simulink model "N3Z_tonetestprevious"  (R2014b)
settings: Solver=ode3  SolverMode=SingleTasking  StartTime=0.0  StopTime=1e-4  FixedStep=fpgaclk  RelTol=1e-3
PreLoadFcn:
  | %fpgaclk=1/32.768e6
  | fpgaclk=1/49.162e6
  | 
  | SerialData=[1,zeros(1,11),1,0,0,1]
  | load ../N3workingG/window
  | win=win';  %Go back to using flatter and wider windowed sync function
  | %load ../N3workingG/hanning    %use Hahn window
  | 
  | load ../N3workingG/PREemphasis   %For pre-empasis and deemphasis FIRs
  | 
  | %LUT3=xls2LUT2('../IQI_Qdemod.xls'); LUT3
  | load ../N3workingG/LUT3
  | load ../N3workingG/FIRiq2
  | % xls2LUT
  | 
  | GetProgFiles
  | 
  | PinAssignments    %Get Pin references for TE0722
  | 
  | 
  | 
  | 
  | 
  | %LCD
  | LCDdata=[LCD_D7,LCD_D6,LCD_D5,LCD_D4,LCD_D3,LCD_D2,LCD_D1,LCD_D0] %Note MSB...LSB!
  | LCDctrl=[LCD_E,LCD_RW,LCD_RS];
  | 
  | %for RS232 on pins 3 and 5 of USBB
  | 
  | %BT chip connections for WT12
  | 
  | RX_BT=RXD
  | TX_BT=TXD
  | 
  | RST_BB=RES
  | 
  | %PCMC=PCMC
  | %PCMS=PCMS
  | %PCMI=PCMI
  | %PCMO=PCMO
  | 
  | %Aliases:
  | SRDBT=PCMI
  | STDBT=PCMO
  | SCLK_BT=PCMC
  | SFS_BT=PCMS
  | 
  | %ADC control
  | 
  | %SDOA=SDOA
  | %SDOB=SDOB
  | %SCK=SCK
  | CONV=Csbar
  | CAL=Cal
  | 
  | ADC_G=[ADC_G3,ADC_G2,ADC_G1,ADC_G0]
  | %PD settings hard coded now
  | 
  | %%%%%%
  | TX_LOW=TX_Low
  | ... (+11 lines)
StartFcn:
  | SerialData=[1,zeros(1,11),1,0,0,1]
values from neighbouring files (symbols this model uses):
  ADC_G0 = {'P10'}    [PinAssignments.m]
  ADC_G1 = {'P11'}    [PinAssignments.m]
  ADC_G2 = {'N14'}    [PinAssignments.m]
  ADC_G3 = {'M11'}    [PinAssignments.m]
  Cal = {'L12'}    [PinAssignments.m]
  Csbar = {'M12'}    [PinAssignments.m]
  LCD_D0 = {'J13'}    [PinAssignments.m]
  LCD_D1 = {'J14'}    [PinAssignments.m]
  LCD_D2 = {'F15'}    [PinAssignments.m]
  LCD_D3 = {'H14'}    [PinAssignments.m]
  LCD_D4 = {'G12'}    [PinAssignments.m]
  LCD_D5 = {'L15'}    [PinAssignments.m]
  LCD_D6 = {'M14'}    [PinAssignments.m]
  LCD_D7 = {'K15'}    [PinAssignments.m]
  PCMC = {'H11'}    [PinAssignments.m]
  PCMI = {'H12'}    [PinAssignments.m]
  PCMO = {'N13'}    [PinAssignments.m]
  PCMS = {'M10'}    [PinAssignments.m]
  RES = {'G11'}    [PinAssignments.m]
  RXD = {'H13'}    [PinAssignments.m]
  TX_Low = {'P15'}    [PinAssignments.m]
  TXD = {'P13'}    [PinAssignments.m]
undefined symbols (not defined in the file or in its folder): AXI4, FIRRX, FIRTX, Lite
libraries: xbsIndex_r4 x1250, MyFunctions x43
(part 7 of 10)

== system N3Z_tonetestprevious/DSProcessor1/OutputRegister/Subsystem11 ==
  Data : Inport
  PortId : Inport  Port=2
  Write : Inport  Port=3
  Logical : xbsIndex_r4/Logical  logical_function=AND  inputs=2  en=off  latency=0  precision=Full  arith_type=Unsigned  n_bits=8  bin_pt=2  align_bp=on  dbl_ovrd=off  block_type=logical
      settings: xl_area=[1 0 0 1 0 0 0]  block_version=VER_STRING_GOES_HERE
  PortAddress : xbsIndex_r4/Constant  const=11  gui_display_data_type=Fixed-point  arith_type=Unsigned  n_bits=8  bin_pt=0  preci_type=Single  exp_width=8  frac_width=24  explicit_period=on  period=fpgaclk  equ=P=C  opselect=C  inp2=PCIN>>17  opr=+  inp1=P  carry=CIN  dbl_ovrd=off  block_type=constant
      settings: block_version=VER_STRING_GOES_HERE
  Register1 : xbsIndex_r4/Register  init=151  rst=off  en=on  dbl_ovrd=off  block_type=register
      settings: xl_area=[4 8 0 0 0 0 0]  block_version=VER_STRING_GOES_HERE
  Relational1 : xbsIndex_r4/Relational  mode=a=b  op_type=Bool  en=off  latency=0  dbl_ovrd=off  block_type=relational
      settings: xl_area=[2 0 0 4 0 0 0]  block_version=VER_STRING_GOES_HERE
  LatchedData : Outport
  wires:
  Relational1/1 -> Logical/1
  Logical/1 -> Register1/2
  PortAddress/1 -> Relational1/2
  Data/1 -> Register1/1
  PortId/1 -> Relational1/1
  Write/1 -> Logical/2
  Register1/1 -> LatchedData/1

== system N3Z_tonetestprevious/DSProcessor1/OutputRegister/Subsystem12 ==
  Data : Inport
  PortId : Inport  Port=2
  Write : Inport  Port=3
  Logical : xbsIndex_r4/Logical  logical_function=AND  inputs=2  en=off  latency=0  precision=Full  arith_type=Unsigned  n_bits=8  bin_pt=2  align_bp=on  dbl_ovrd=off  block_type=logical
      settings: xl_area=[1 0 0 1 0 0 0]  block_version=VER_STRING_GOES_HERE
  PortAddress : xbsIndex_r4/Constant  const=12  gui_display_data_type=Fixed-point  arith_type=Unsigned  n_bits=8  bin_pt=0  preci_type=Single  exp_width=8  frac_width=24  explicit_period=on  period=fpgaclk  equ=P=C  opselect=C  inp2=PCIN>>17  opr=+  inp1=P  carry=CIN  dbl_ovrd=off  block_type=constant
      settings: block_version=VER_STRING_GOES_HERE
  Register1 : xbsIndex_r4/Register  init=151  rst=off  en=on  dbl_ovrd=off  block_type=register
      settings: xl_area=[4 8 0 0 0 0 0]  block_version=VER_STRING_GOES_HERE
  Relational1 : xbsIndex_r4/Relational  mode=a=b  op_type=Bool  en=off  latency=0  dbl_ovrd=off  block_type=relational
      settings: xl_area=[2 0 0 4 0 0 0]  block_version=VER_STRING_GOES_HERE
  LatchedData : Outport
  Ack_Fifo : Outport  Port=2
  wires:
  Relational1/1 -> Logical/1
  Logical/1 -> Register1/2, Ack_Fifo/1
  PortAddress/1 -> Relational1/2
  Data/1 -> Register1/1
  PortId/1 -> Relational1/1
  Write/1 -> Logical/2
  Register1/1 -> LatchedData/1

== system N3Z_tonetestprevious/DSProcessor1/OutputRegister/Subsystem13 ==
  Data : Inport
  PortId : Inport  Port=2
  Write : Inport  Port=3
  Logical : xbsIndex_r4/Logical  logical_function=AND  inputs=2  en=off  latency=0  precision=Full  arith_type=Unsigned  n_bits=8  bin_pt=2  align_bp=on  dbl_ovrd=off  block_type=logical
      settings: xl_area=[1 0 0 1 0 0 0]  block_version=VER_STRING_GOES_HERE
  PortAddress : xbsIndex_r4/Constant  const=13  gui_display_data_type=Fixed-point  arith_type=Unsigned  n_bits=8  bin_pt=0  preci_type=Single  exp_width=8  frac_width=24  explicit_period=on  period=fpgaclk  equ=P=C  opselect=C  inp2=PCIN>>17  opr=+  inp1=P  carry=CIN  dbl_ovrd=off  block_type=constant
      settings: block_version=VER_STRING_GOES_HERE
  Register1 : xbsIndex_r4/Register  init=0  rst=off  en=on  dbl_ovrd=off  block_type=register
      settings: xl_area=[4 8 0 0 0 0 0]  block_version=VER_STRING_GOES_HERE
  Relational1 : xbsIndex_r4/Relational  mode=a=b  op_type=Bool  en=off  latency=0  dbl_ovrd=off  block_type=relational
      settings: xl_area=[2 0 0 4 0 0 0]  block_version=VER_STRING_GOES_HERE
  LatchedData : Outport
  NewValue : Outport  Port=2
  wires:
  Relational1/1 -> Logical/1
  Logical/1 -> Register1/2, NewValue/1
  PortAddress/1 -> Relational1/2
  Data/1 -> Register1/1
  PortId/1 -> Relational1/1
  Write/1 -> Logical/2
  Register1/1 -> LatchedData/1

== system N3Z_tonetestprevious/DSProcessor1/OutputRegister/Subsystem14 ==
  Data : Inport
  PortId : Inport  Port=2
  Write : Inport  Port=3
  Logical : xbsIndex_r4/Logical  logical_function=AND  inputs=2  en=off  latency=0  precision=Full  arith_type=Unsigned  n_bits=8  bin_pt=2  align_bp=on  dbl_ovrd=off  block_type=logical
      settings: xl_area=[1 0 0 1 0 0 0]  block_version=VER_STRING_GOES_HERE
  PortAddress : xbsIndex_r4/Constant  const=14  gui_display_data_type=Fixed-point  arith_type=Unsigned  n_bits=8  bin_pt=0  preci_type=Single  exp_width=8  frac_width=24  explicit_period=on  period=fpgaclk  equ=P=C  opselect=C  inp2=PCIN>>17  opr=+  inp1=P  carry=CIN  dbl_ovrd=off  block_type=constant
      settings: block_version=VER_STRING_GOES_HERE
  Register1 : xbsIndex_r4/Register  init=0  rst=off  en=on  dbl_ovrd=off  block_type=register
      settings: xl_area=[4 8 0 0 0 0 0]  block_version=VER_STRING_GOES_HERE
  Relational1 : xbsIndex_r4/Relational  mode=a=b  op_type=Bool  en=off  latency=0  dbl_ovrd=off  block_type=relational
      settings: xl_area=[2 0 0 4 0 0 0]  block_version=VER_STRING_GOES_HERE
  LatchedData : Outport
  wires:
  Relational1/1 -> Logical/1
  Logical/1 -> Register1/2
  PortAddress/1 -> Relational1/2
  Data/1 -> Register1/1
  PortId/1 -> Relational1/1
  Write/1 -> Logical/2
  Register1/1 -> LatchedData/1

== system N3Z_tonetestprevious/DSProcessor1/OutputRegister/Subsystem15 ==
  Data : Inport
  PortId : Inport  Port=2
  Write : Inport  Port=3
  Logical : xbsIndex_r4/Logical  logical_function=AND  inputs=2  en=off  latency=0  precision=Full  arith_type=Unsigned  n_bits=8  bin_pt=2  align_bp=on  dbl_ovrd=off  block_type=logical
      settings: xl_area=[1 0 0 1 0 0 0]  block_version=VER_STRING_GOES_HERE
  PortAddress : xbsIndex_r4/Constant  const=15  gui_display_data_type=Fixed-point  arith_type=Unsigned  n_bits=8  bin_pt=0  preci_type=Single  exp_width=8  frac_width=24  explicit_period=on  period=fpgaclk  equ=P=C  opselect=C  inp2=PCIN>>17  opr=+  inp1=P  carry=CIN  dbl_ovrd=off  block_type=constant
      settings: block_version=VER_STRING_GOES_HERE
  Register1 : xbsIndex_r4/Register  init=0  rst=off  en=on  dbl_ovrd=off  block_type=register
      settings: xl_area=[4 8 0 0 0 0 0]  block_version=VER_STRING_GOES_HERE
  Relational1 : xbsIndex_r4/Relational  mode=a=b  op_type=Bool  en=off  latency=0  dbl_ovrd=off  block_type=relational
      settings: xl_area=[2 0 0 4 0 0 0]  block_version=VER_STRING_GOES_HERE
  LatchedData : Outport
  wires:
  Relational1/1 -> Logical/1
  Logical/1 -> Register1/2
  PortAddress/1 -> Relational1/2
  Data/1 -> Register1/1
  PortId/1 -> Relational1/1
  Write/1 -> Logical/2
  Register1/1 -> LatchedData/1

== system N3Z_tonetestprevious/DSProcessor1/OutputRegister/Subsystem16 ==
  Data : Inport
  PortId : Inport  Port=2
  Write : Inport  Port=3
  Logical : xbsIndex_r4/Logical  logical_function=AND  inputs=2  en=off  latency=0  precision=Full  arith_type=Unsigned  n_bits=8  bin_pt=2  align_bp=on  dbl_ovrd=off  block_type=logical
      settings: xl_area=[1 0 0 1 0 0 0]  block_version=VER_STRING_GOES_HERE
  PortAddress : xbsIndex_r4/Constant  const=16  gui_display_data_type=Fixed-point  arith_type=Unsigned  n_bits=8  bin_pt=0  preci_type=Single  exp_width=8  frac_width=24  explicit_period=on  period=fpgaclk  equ=P=C  opselect=C  inp2=PCIN>>17  opr=+  inp1=P  carry=CIN  dbl_ovrd=off  block_type=constant
      settings: block_version=VER_STRING_GOES_HERE
  Register1 : xbsIndex_r4/Register  init=0  rst=off  en=on  dbl_ovrd=off  block_type=register
      settings: xl_area=[4 8 0 0 0 0 0]  block_version=VER_STRING_GOES_HERE
  Relational1 : xbsIndex_r4/Relational  mode=a=b  op_type=Bool  en=off  latency=0  dbl_ovrd=off  block_type=relational
      settings: xl_area=[2 0 0 4 0 0 0]  block_version=VER_STRING_GOES_HERE
  LatchedData : Outport
  wires:
  Relational1/1 -> Logical/1
  Logical/1 -> Register1/2
  PortAddress/1 -> Relational1/2
  Data/1 -> Register1/1
  PortId/1 -> Relational1/1
  Write/1 -> Logical/2
  Register1/1 -> LatchedData/1

== system N3Z_tonetestprevious/DSProcessor1/OutputRegister/Subsystem17 ==
  Data : Inport
  PortId : Inport  Port=2
  Write : Inport  Port=3
  Logical : xbsIndex_r4/Logical  logical_function=AND  inputs=2  en=off  latency=0  precision=Full  arith_type=Unsigned  n_bits=8  bin_pt=2  align_bp=on  dbl_ovrd=off  block_type=logical
      settings: xl_area=[1 0 0 1 0 0 0]  block_version=VER_STRING_GOES_HERE
  PortAddress : xbsIndex_r4/Constant  const=17  gui_display_data_type=Fixed-point  arith_type=Unsigned  n_bits=8  bin_pt=0  preci_type=Single  exp_width=8  frac_width=24  explicit_period=on  period=fpgaclk  equ=P=C  opselect=C  inp2=PCIN>>17  opr=+  inp1=P  carry=CIN  dbl_ovrd=off  block_type=constant
      settings: block_version=VER_STRING_GOES_HERE
  Register1 : xbsIndex_r4/Register  init=1  rst=off  en=on  dbl_ovrd=off  block_type=register
      settings: xl_area=[4 8 0 0 0 0 0]  block_version=VER_STRING_GOES_HERE
  Relational1 : xbsIndex_r4/Relational  mode=a=b  op_type=Bool  en=off  latency=0  dbl_ovrd=off  block_type=relational
      settings: xl_area=[2 0 0 4 0 0 0]  block_version=VER_STRING_GOES_HERE
  LatchedData : Outport
  wires:
  Relational1/1 -> Logical/1
  Logical/1 -> Register1/2
  PortAddress/1 -> Relational1/2
  Data/1 -> Register1/1
  PortId/1 -> Relational1/1
  Write/1 -> Logical/2
  Register1/1 -> LatchedData/1

== system N3Z_tonetestprevious/DSProcessor1/OutputRegister/Subsystem18 ==
  Data : Inport
  PortId : Inport  Port=2
  Write : Inport  Port=3
  Logical : xbsIndex_r4/Logical  logical_function=AND  inputs=2  en=off  latency=0  precision=Full  arith_type=Unsigned  n_bits=8  bin_pt=2  align_bp=on  dbl_ovrd=off  block_type=logical
      settings: xl_area=[1 0 0 1 0 0 0]  block_version=VER_STRING_GOES_HERE
  PortAddress : xbsIndex_r4/Constant  const=18  gui_display_data_type=Fixed-point  arith_type=Unsigned  n_bits=8  bin_pt=0  preci_type=Single  exp_width=8  frac_width=24  explicit_period=on  period=fpgaclk  equ=P=C  opselect=C  inp2=PCIN>>17  opr=+  inp1=P  carry=CIN  dbl_ovrd=off  block_type=constant
      settings: block_version=VER_STRING_GOES_HERE
  Register1 : xbsIndex_r4/Register  init=0  rst=off  en=on  dbl_ovrd=off  block_type=register
      settings: xl_area=[4 8 0 0 0 0 0]  block_version=VER_STRING_GOES_HERE
  Relational1 : xbsIndex_r4/Relational  mode=a=b  op_type=Bool  en=off  latency=0  dbl_ovrd=off  block_type=relational
      settings: xl_area=[2 0 0 4 0 0 0]  block_version=VER_STRING_GOES_HERE
  LatchedData : Outport
  wires:
  Relational1/1 -> Logical/1
  Logical/1 -> Register1/2
  PortAddress/1 -> Relational1/2
  Data/1 -> Register1/1
  PortId/1 -> Relational1/1
  Write/1 -> Logical/2
  Register1/1 -> LatchedData/1

== system N3Z_tonetestprevious/DSProcessor1/OutputRegister/Subsystem19 ==
  Data : Inport
  PortId : Inport  Port=2
  Write : Inport  Port=3
  Logical : xbsIndex_r4/Logical  logical_function=AND  inputs=2  en=off  latency=0  precision=Full  arith_type=Unsigned  n_bits=8  bin_pt=2  align_bp=on  dbl_ovrd=off  block_type=logical
      settings: xl_area=[1 0 0 1 0 0 0]  block_version=VER_STRING_GOES_HERE
  PortAddress : xbsIndex_r4/Constant  const=19  gui_display_data_type=Fixed-point  arith_type=Unsigned  n_bits=8  bin_pt=0  preci_type=Single  exp_width=8  frac_width=24  explicit_period=on  period=fpgaclk  equ=P=C  opselect=C  inp2=PCIN>>17  opr=+  inp1=P  carry=CIN  dbl_ovrd=off  block_type=constant
      settings: block_version=VER_STRING_GOES_HERE
  Register1 : xbsIndex_r4/Register  init=0  rst=off  en=on  dbl_ovrd=off  block_type=register
      settings: xl_area=[4 8 0 0 0 0 0]  block_version=VER_STRING_GOES_HERE
  Relational1 : xbsIndex_r4/Relational  mode=a=b  op_type=Bool  en=off  latency=0  dbl_ovrd=off  block_type=relational
      settings: xl_area=[2 0 0 4 0 0 0]  block_version=VER_STRING_GOES_HERE
  LatchedData : Outport
  wires:
  Relational1/1 -> Logical/1
  Logical/1 -> Register1/2
  PortAddress/1 -> Relational1/2
  Data/1 -> Register1/1
  PortId/1 -> Relational1/1
  Write/1 -> Logical/2
  Register1/1 -> LatchedData/1

== system N3Z_tonetestprevious/DSProcessor1/OutputRegister/Subsystem2 ==
  Data : Inport
  PortId : Inport  Port=2
  Write : Inport  Port=3
  Logical : xbsIndex_r4/Logical  logical_function=AND  inputs=2  en=off  latency=0  precision=Full  arith_type=Unsigned  n_bits=8  bin_pt=2  align_bp=on  dbl_ovrd=off  block_type=logical
      settings: xl_area=[1 0 0 1 0 0 0]  block_version=VER_STRING_GOES_HERE
  PortAddress : xbsIndex_r4/Constant  const=3  gui_display_data_type=Fixed-point  arith_type=Unsigned  n_bits=8  bin_pt=0  preci_type=Single  exp_width=8  frac_width=24  explicit_period=on  period=fpgaclk  equ=P=C  opselect=C  inp2=PCIN>>17  opr=+  inp1=P  carry=CIN  dbl_ovrd=off  block_type=constant
      settings: block_version=VER_STRING_GOES_HERE
  Register1 : xbsIndex_r4/Register  init=0  rst=off  en=on  dbl_ovrd=off  block_type=register
      settings: xl_area=[4 8 0 0 0 0 0]  block_version=VER_STRING_GOES_HERE
  Relational1 : xbsIndex_r4/Relational  mode=a=b  op_type=Bool  en=off  latency=0  dbl_ovrd=off  block_type=relational
      settings: xl_area=[2 0 0 4 0 0 0]  block_version=VER_STRING_GOES_HERE
  LatchedData : Outport
  Strobe : Outport  Port=2
  wires:
  Relational1/1 -> Logical/1
  Logical/1 -> Register1/2, Strobe/1
  PortAddress/1 -> Relational1/2
  Data/1 -> Register1/1
  PortId/1 -> Relational1/1
  Write/1 -> Logical/2
  Register1/1 -> LatchedData/1

== system N3Z_tonetestprevious/DSProcessor1/OutputRegister/Subsystem20 ==
  Data : Inport
  PortId : Inport  Port=2
  Write : Inport  Port=3
  Logical : xbsIndex_r4/Logical  logical_function=AND  inputs=2  en=off  latency=0  precision=Full  arith_type=Unsigned  n_bits=8  bin_pt=2  align_bp=on  dbl_ovrd=off  block_type=logical
      settings: xl_area=[1 0 0 1 0 0 0]  block_version=VER_STRING_GOES_HERE
  PortAddress : xbsIndex_r4/Constant  const=20  gui_display_data_type=Fixed-point  arith_type=Unsigned  n_bits=8  bin_pt=0  preci_type=Single  exp_width=8  frac_width=24  explicit_period=on  period=fpgaclk  equ=P=C  opselect=C  inp2=PCIN>>17  opr=+  inp1=P  carry=CIN  dbl_ovrd=off  block_type=constant
      settings: block_version=VER_STRING_GOES_HERE
  Register1 : xbsIndex_r4/Register  init=0  rst=off  en=on  dbl_ovrd=off  block_type=register
      settings: xl_area=[4 8 0 0 0 0 0]  block_version=VER_STRING_GOES_HERE
  Relational1 : xbsIndex_r4/Relational  mode=a=b  op_type=Bool  en=off  latency=0  dbl_ovrd=off  block_type=relational
      settings: xl_area=[2 0 0 4 0 0 0]  block_version=VER_STRING_GOES_HERE
  LatchedData : Outport
  wires:
  Relational1/1 -> Logical/1
  Logical/1 -> Register1/2
  PortAddress/1 -> Relational1/2
  Data/1 -> Register1/1
  PortId/1 -> Relational1/1
  Write/1 -> Logical/2
  Register1/1 -> LatchedData/1

== system N3Z_tonetestprevious/DSProcessor1/OutputRegister/Subsystem21 ==
  Data : Inport
  PortId : Inport  Port=2
  Write : Inport  Port=3
  Logical : xbsIndex_r4/Logical  logical_function=AND  inputs=2  en=off  latency=0  precision=Full  arith_type=Unsigned  n_bits=8  bin_pt=2  align_bp=on  dbl_ovrd=off  block_type=logical
      settings: xl_area=[1 0 0 1 0 0 0]  block_version=VER_STRING_GOES_HERE
  PortAddress : xbsIndex_r4/Constant  const=21  gui_display_data_type=Fixed-point  arith_type=Unsigned  n_bits=8  bin_pt=0  preci_type=Single  exp_width=8  frac_width=24  explicit_period=on  period=fpgaclk  equ=P=C  opselect=C  inp2=PCIN>>17  opr=+  inp1=P  carry=CIN  dbl_ovrd=off  block_type=constant
      settings: block_version=VER_STRING_GOES_HERE
  Register1 : xbsIndex_r4/Register  init=0  rst=off  en=on  dbl_ovrd=off  block_type=register
      settings: xl_area=[4 8 0 0 0 0 0]  block_version=VER_STRING_GOES_HERE
  Relational1 : xbsIndex_r4/Relational  mode=a=b  op_type=Bool  en=off  latency=0  dbl_ovrd=off  block_type=relational
      settings: xl_area=[2 0 0 4 0 0 0]  block_version=VER_STRING_GOES_HERE
  LatchedData : Outport
  wires:
  Relational1/1 -> Logical/1
  Logical/1 -> Register1/2
  PortAddress/1 -> Relational1/2
  Data/1 -> Register1/1
  PortId/1 -> Relational1/1
  Write/1 -> Logical/2
  Register1/1 -> LatchedData/1

== system N3Z_tonetestprevious/DSProcessor1/OutputRegister/Subsystem22 ==
  Data : Inport
  PortId : Inport  Port=2
  Write : Inport  Port=3
  Logical : xbsIndex_r4/Logical  logical_function=AND  inputs=2  en=off  latency=0  precision=Full  arith_type=Unsigned  n_bits=8  bin_pt=2  align_bp=on  dbl_ovrd=off  block_type=logical
      settings: xl_area=[1 0 0 1 0 0 0]  block_version=VER_STRING_GOES_HERE
  PortAddress : xbsIndex_r4/Constant  const=22  gui_display_data_type=Fixed-point  arith_type=Unsigned  n_bits=8  bin_pt=0  preci_type=Single  exp_width=8  frac_width=24  explicit_period=on  period=fpgaclk  equ=P=C  opselect=C  inp2=PCIN>>17  opr=+  inp1=P  carry=CIN  dbl_ovrd=off  block_type=constant
      settings: block_version=VER_STRING_GOES_HERE
  Register1 : xbsIndex_r4/Register  init=0  rst=off  en=on  dbl_ovrd=off  block_type=register
      settings: xl_area=[4 8 0 0 0 0 0]  block_version=VER_STRING_GOES_HERE
  Relational1 : xbsIndex_r4/Relational  mode=a=b  op_type=Bool  en=off  latency=0  dbl_ovrd=off  block_type=relational
      settings: xl_area=[2 0 0 4 0 0 0]  block_version=VER_STRING_GOES_HERE
  LatchedData : Outport
  wires:
  Relational1/1 -> Logical/1
  Logical/1 -> Register1/2
  PortAddress/1 -> Relational1/2
  Data/1 -> Register1/1
  PortId/1 -> Relational1/1
  Write/1 -> Logical/2
  Register1/1 -> LatchedData/1

== system N3Z_tonetestprevious/DSProcessor1/OutputRegister/Subsystem23 ==
  Data : Inport
  PortId : Inport  Port=2
  Write : Inport  Port=3
  Logical : xbsIndex_r4/Logical  logical_function=AND  inputs=2  en=off  latency=0  precision=Full  arith_type=Unsigned  n_bits=8  bin_pt=2  align_bp=on  dbl_ovrd=off  block_type=logical
      settings: xl_area=[1 0 0 1 0 0 0]  block_version=VER_STRING_GOES_HERE
  PortAddress : xbsIndex_r4/Constant  const=23  gui_display_data_type=Fixed-point  arith_type=Unsigned  n_bits=8  bin_pt=0  preci_type=Single  exp_width=8  frac_width=24  explicit_period=on  period=fpgaclk  equ=P=C  opselect=C  inp2=PCIN>>17  opr=+  inp1=P  carry=CIN  dbl_ovrd=off  block_type=constant
      settings: block_version=VER_STRING_GOES_HERE
  Register1 : xbsIndex_r4/Register  init=0  rst=off  en=on  dbl_ovrd=off  block_type=register
      settings: xl_area=[4 8 0 0 0 0 0]  block_version=VER_STRING_GOES_HERE
  Relational1 : xbsIndex_r4/Relational  mode=a=b  op_type=Bool  en=off  latency=0  dbl_ovrd=off  block_type=relational
      settings: xl_area=[2 0 0 4 0 0 0]  block_version=VER_STRING_GOES_HERE
  LatchedData : Outport
  wires:
  Relational1/1 -> Logical/1
  Logical/1 -> Register1/2
  PortAddress/1 -> Relational1/2
  Data/1 -> Register1/1
  PortId/1 -> Relational1/1
  Write/1 -> Logical/2
  Register1/1 -> LatchedData/1

== system N3Z_tonetestprevious/DSProcessor1/OutputRegister/Subsystem24 ==
  Data : Inport
  PortId : Inport  Port=2
  Write : Inport  Port=3
  Logical : xbsIndex_r4/Logical  logical_function=AND  inputs=2  en=off  latency=0  precision=Full  arith_type=Unsigned  n_bits=8  bin_pt=2  align_bp=on  dbl_ovrd=off  block_type=logical
      settings: xl_area=[1 0 0 1 0 0 0]  block_version=VER_STRING_GOES_HERE
  PortAddress : xbsIndex_r4/Constant  const=24  gui_display_data_type=Fixed-point  arith_type=Unsigned  n_bits=8  bin_pt=0  preci_type=Single  exp_width=8  frac_width=24  explicit_period=on  period=fpgaclk  equ=P=C  opselect=C  inp2=PCIN>>17  opr=+  inp1=P  carry=CIN  dbl_ovrd=off  block_type=constant
      settings: block_version=VER_STRING_GOES_HERE
  Register1 : xbsIndex_r4/Register  init=0  rst=off  en=on  dbl_ovrd=off  block_type=register
      settings: xl_area=[4 8 0 0 0 0 0]  block_version=VER_STRING_GOES_HERE
  Relational1 : xbsIndex_r4/Relational  mode=a=b  op_type=Bool  en=off  latency=0  dbl_ovrd=off  block_type=relational
      settings: xl_area=[2 0 0 4 0 0 0]  block_version=VER_STRING_GOES_HERE
  LatchedData : Outport
  wires:
  Relational1/1 -> Logical/1
  Logical/1 -> Register1/2
  PortAddress/1 -> Relational1/2
  Data/1 -> Register1/1
  PortId/1 -> Relational1/1
  Write/1 -> Logical/2
  Register1/1 -> LatchedData/1

== system N3Z_tonetestprevious/DSProcessor1/OutputRegister/Subsystem25 ==
  Data : Inport
  PortId : Inport  Port=2
  Write : Inport  Port=3
  Logical : xbsIndex_r4/Logical  logical_function=AND  inputs=2  en=off  latency=0  precision=Full  arith_type=Unsigned  n_bits=8  bin_pt=2  align_bp=on  dbl_ovrd=off  block_type=logical
      settings: xl_area=[1 0 0 1 0 0 0]  block_version=VER_STRING_GOES_HERE
  PortAddress : xbsIndex_r4/Constant  const=25  gui_display_data_type=Fixed-point  arith_type=Unsigned  n_bits=8  bin_pt=0  preci_type=Single  exp_width=8  frac_width=24  explicit_period=on  period=fpgaclk  equ=P=C  opselect=C  inp2=PCIN>>17  opr=+  inp1=P  carry=CIN  dbl_ovrd=off  block_type=constant
      settings: block_version=VER_STRING_GOES_HERE
  Register1 : xbsIndex_r4/Register  init=0  rst=off  en=on  dbl_ovrd=off  block_type=register
      settings: xl_area=[4 8 0 0 0 0 0]  block_version=VER_STRING_GOES_HERE
  Relational1 : xbsIndex_r4/Relational  mode=a=b  op_type=Bool  en=off  latency=0  dbl_ovrd=off  block_type=relational
      settings: xl_area=[2 0 0 4 0 0 0]  block_version=VER_STRING_GOES_HERE
  LatchedData : Outport
  wires:
  Relational1/1 -> Logical/1
  Logical/1 -> Register1/2
  PortAddress/1 -> Relational1/2
  Data/1 -> Register1/1
  PortId/1 -> Relational1/1
  Write/1 -> Logical/2
  Register1/1 -> LatchedData/1

== system N3Z_tonetestprevious/DSProcessor1/OutputRegister/Subsystem26 ==
  Data : Inport
  PortId : Inport  Port=2
  Write : Inport  Port=3
  Logical : xbsIndex_r4/Logical  logical_function=AND  inputs=2  en=off  latency=0  precision=Full  arith_type=Unsigned  n_bits=8  bin_pt=2  align_bp=on  dbl_ovrd=off  block_type=logical
      settings: xl_area=[1 0 0 1 0 0 0]  block_version=VER_STRING_GOES_HERE
  PortAddress : xbsIndex_r4/Constant  const=26  gui_display_data_type=Fixed-point  arith_type=Unsigned  n_bits=8  bin_pt=0  preci_type=Single  exp_width=8  frac_width=24  explicit_period=on  period=fpgaclk  equ=P=C  opselect=C  inp2=PCIN>>17  opr=+  inp1=P  carry=CIN  dbl_ovrd=off  block_type=constant
      settings: block_version=VER_STRING_GOES_HERE
  Register1 : xbsIndex_r4/Register  init=0  rst=off  en=on  dbl_ovrd=off  block_type=register
      settings: xl_area=[4 8 0 0 0 0 0]  block_version=VER_STRING_GOES_HERE
  Relational1 : xbsIndex_r4/Relational  mode=a=b  op_type=Bool  en=off  latency=0  dbl_ovrd=off  block_type=relational
      settings: xl_area=[2 0 0 4 0 0 0]  block_version=VER_STRING_GOES_HERE
  LatchedData : Outport
  wires:
  Relational1/1 -> Logical/1
  Logical/1 -> Register1/2
  PortAddress/1 -> Relational1/2
  Data/1 -> Register1/1
  PortId/1 -> Relational1/1
  Write/1 -> Logical/2
  Register1/1 -> LatchedData/1

== system N3Z_tonetestprevious/DSProcessor1/OutputRegister/Subsystem27 ==
  Data : Inport
  PortId : Inport  Port=2
  Write : Inport  Port=3
  Logical : xbsIndex_r4/Logical  logical_function=AND  inputs=2  en=off  latency=0  precision=Full  arith_type=Unsigned  n_bits=8  bin_pt=2  align_bp=on  dbl_ovrd=off  block_type=logical
      settings: xl_area=[1 0 0 1 0 0 0]  block_version=VER_STRING_GOES_HERE
  PortAddress : xbsIndex_r4/Constant  const=27  gui_display_data_type=Fixed-point  arith_type=Unsigned  n_bits=8  bin_pt=0  preci_type=Single  exp_width=8  frac_width=24  explicit_period=on  period=fpgaclk  equ=P=C  opselect=C  inp2=PCIN>>17  opr=+  inp1=P  carry=CIN  dbl_ovrd=off  block_type=constant
      settings: block_version=VER_STRING_GOES_HERE
  Register1 : xbsIndex_r4/Register  init=0  rst=off  en=on  dbl_ovrd=off  block_type=register
      settings: xl_area=[4 8 0 0 0 0 0]  block_version=VER_STRING_GOES_HERE
  Relational1 : xbsIndex_r4/Relational  mode=a=b  op_type=Bool  en=off  latency=0  dbl_ovrd=off  block_type=relational
      settings: xl_area=[2 0 0 4 0 0 0]  block_version=VER_STRING_GOES_HERE
  LatchedData : Outport
  wires:
  Relational1/1 -> Logical/1
  Logical/1 -> Register1/2
  PortAddress/1 -> Relational1/2
  Data/1 -> Register1/1
  PortId/1 -> Relational1/1
  Write/1 -> Logical/2
  Register1/1 -> LatchedData/1

== system N3Z_tonetestprevious/DSProcessor1/OutputRegister/Subsystem28 ==
  Data : Inport
  PortId : Inport  Port=2
  Write : Inport  Port=3
  Logical : xbsIndex_r4/Logical  logical_function=AND  inputs=2  en=off  latency=0  precision=Full  arith_type=Unsigned  n_bits=8  bin_pt=2  align_bp=on  dbl_ovrd=off  block_type=logical
      settings: xl_area=[1 0 0 1 0 0 0]  block_version=VER_STRING_GOES_HERE
  PortAddress : xbsIndex_r4/Constant  const=28  gui_display_data_type=Fixed-point  arith_type=Unsigned  n_bits=8  bin_pt=0  preci_type=Single  exp_width=8  frac_width=24  explicit_period=on  period=fpgaclk  equ=P=C  opselect=C  inp2=PCIN>>17  opr=+  inp1=P  carry=CIN  dbl_ovrd=off  block_type=constant
      settings: block_version=VER_STRING_GOES_HERE
  Register1 : xbsIndex_r4/Register  init=0  rst=off  en=on  dbl_ovrd=off  block_type=register
      settings: xl_area=[4 8 0 0 0 0 0]  block_version=VER_STRING_GOES_HERE
  Relational1 : xbsIndex_r4/Relational  mode=a=b  op_type=Bool  en=off  latency=0  dbl_ovrd=off  block_type=relational
      settings: xl_area=[2 0 0 4 0 0 0]  block_version=VER_STRING_GOES_HERE
  LatchedData : Outport
  wires:
  Relational1/1 -> Logical/1
  Logical/1 -> Register1/2
  PortAddress/1 -> Relational1/2
  Data/1 -> Register1/1
  PortId/1 -> Relational1/1
  Write/1 -> Logical/2
  Register1/1 -> LatchedData/1

== system N3Z_tonetestprevious/DSProcessor1/OutputRegister/Subsystem3 ==
  Data : Inport
  PortId : Inport  Port=2
  Write : Inport  Port=3
  Logical : xbsIndex_r4/Logical  logical_function=AND  inputs=2  en=off  latency=0  precision=Full  arith_type=Unsigned  n_bits=8  bin_pt=2  align_bp=on  dbl_ovrd=off  block_type=logical
      settings: xl_area=[1 0 0 1 0 0 0]  block_version=VER_STRING_GOES_HERE
  PortAddress : xbsIndex_r4/Constant  const=4  gui_display_data_type=Fixed-point  arith_type=Unsigned  n_bits=8  bin_pt=0  preci_type=Single  exp_width=8  frac_width=24  explicit_period=on  period=fpgaclk  equ=P=C  opselect=C  inp2=PCIN>>17  opr=+  inp1=P  carry=CIN  dbl_ovrd=off  block_type=constant
      settings: block_version=VER_STRING_GOES_HERE
  Register1 : xbsIndex_r4/Register  init=0  rst=off  en=on  dbl_ovrd=off  block_type=register
      settings: xl_area=[4 8 0 0 0 0 0]  block_version=VER_STRING_GOES_HERE
  Relational1 : xbsIndex_r4/Relational  mode=a=b  op_type=Bool  en=off  latency=0  dbl_ovrd=off  block_type=relational
      settings: xl_area=[2 0 0 4 0 0 0]  block_version=VER_STRING_GOES_HERE
  LatchedData : Outport
  wires:
  Relational1/1 -> Logical/1
  Logical/1 -> Register1/2
  PortAddress/1 -> Relational1/2
  Data/1 -> Register1/1
  PortId/1 -> Relational1/1
  Write/1 -> Logical/2
  Register1/1 -> LatchedData/1

== system N3Z_tonetestprevious/DSProcessor1/OutputRegister/Subsystem4 ==
  Data : Inport
  PortId : Inport  Port=2
  Write : Inport  Port=3
  Logical : xbsIndex_r4/Logical  logical_function=AND  inputs=2  en=off  latency=0  precision=Full  arith_type=Unsigned  n_bits=8  bin_pt=2  align_bp=on  dbl_ovrd=off  block_type=logical
      settings: xl_area=[1 0 0 1 0 0 0]  block_version=VER_STRING_GOES_HERE
  PortAddress : xbsIndex_r4/Constant  const=5  gui_display_data_type=Fixed-point  arith_type=Unsigned  n_bits=8  bin_pt=0  preci_type=Single  exp_width=8  frac_width=24  explicit_period=on  period=fpgaclk  equ=P=C  opselect=C  inp2=PCIN>>17  opr=+  inp1=P  carry=CIN  dbl_ovrd=off  block_type=constant
      settings: block_version=VER_STRING_GOES_HERE
  Register1 : xbsIndex_r4/Register  init=0  rst=off  en=on  dbl_ovrd=off  block_type=register
      settings: xl_area=[4 8 0 0 0 0 0]  block_version=VER_STRING_GOES_HERE
  Relational1 : xbsIndex_r4/Relational  mode=a=b  op_type=Bool  en=off  latency=0  dbl_ovrd=off  block_type=relational
      settings: xl_area=[2 0 0 4 0 0 0]  block_version=VER_STRING_GOES_HERE
  LatchedData : Outport
  wires:
  Relational1/1 -> Logical/1
  Logical/1 -> Register1/2
  PortAddress/1 -> Relational1/2
  Data/1 -> Register1/1
  PortId/1 -> Relational1/1
  Write/1 -> Logical/2
  Register1/1 -> LatchedData/1

== system N3Z_tonetestprevious/DSProcessor1/OutputRegister/Subsystem5 ==
  Data : Inport
  PortId : Inport  Port=2
  Write : Inport  Port=3
  Logical : xbsIndex_r4/Logical  logical_function=AND  inputs=2  en=off  latency=0  precision=Full  arith_type=Unsigned  n_bits=8  bin_pt=2  align_bp=on  dbl_ovrd=off  block_type=logical
      settings: xl_area=[1 0 0 1 0 0 0]  block_version=VER_STRING_GOES_HERE
  PortAddress : xbsIndex_r4/Constant  const=6  gui_display_data_type=Fixed-point  arith_type=Unsigned  n_bits=8  bin_pt=0  preci_type=Single  exp_width=8  frac_width=24  explicit_period=on  period=fpgaclk  equ=P=C  opselect=C  inp2=PCIN>>17  opr=+  inp1=P  carry=CIN  dbl_ovrd=off  block_type=constant
      settings: block_version=VER_STRING_GOES_HERE
  Register1 : xbsIndex_r4/Register  init=0  rst=off  en=on  dbl_ovrd=off  block_type=register
      settings: xl_area=[4 8 0 0 0 0 0]  block_version=VER_STRING_GOES_HERE
  Relational1 : xbsIndex_r4/Relational  mode=a=b  op_type=Bool  en=off  latency=0  dbl_ovrd=off  block_type=relational
      settings: xl_area=[2 0 0 4 0 0 0]  block_version=VER_STRING_GOES_HERE
  LatchedData : Outport
  wires:
  Relational1/1 -> Logical/1
  Logical/1 -> Register1/2
  PortAddress/1 -> Relational1/2
  Data/1 -> Register1/1
  PortId/1 -> Relational1/1
  Write/1 -> Logical/2
  Register1/1 -> LatchedData/1

== system N3Z_tonetestprevious/DSProcessor1/OutputRegister/Subsystem6 ==
  Data : Inport
  PortId : Inport  Port=2
  Write : Inport  Port=3
  Logical : xbsIndex_r4/Logical  logical_function=AND  inputs=2  en=off  latency=0  precision=Full  arith_type=Unsigned  n_bits=8  bin_pt=2  align_bp=on  dbl_ovrd=off  block_type=logical
      settings: xl_area=[1 0 0 1 0 0 0]  block_version=VER_STRING_GOES_HERE
  PortAddress : xbsIndex_r4/Constant  const=7  gui_display_data_type=Fixed-point  arith_type=Unsigned  n_bits=8  bin_pt=0  preci_type=Single  exp_width=8  frac_width=24  explicit_period=on  period=fpgaclk  equ=P=C  opselect=C  inp2=PCIN>>17  opr=+  inp1=P  carry=CIN  dbl_ovrd=off  block_type=constant
      settings: block_version=VER_STRING_GOES_HERE
  Register1 : xbsIndex_r4/Register  init=0  rst=off  en=on  dbl_ovrd=off  block_type=register
      settings: xl_area=[4 8 0 0 0 0 0]  block_version=VER_STRING_GOES_HERE
  Relational1 : xbsIndex_r4/Relational  mode=a=b  op_type=Bool  en=off  latency=0  dbl_ovrd=off  block_type=relational
      settings: xl_area=[2 0 0 4 0 0 0]  block_version=VER_STRING_GOES_HERE
  LatchedData : Outport
  wires:
  Relational1/1 -> Logical/1
  Logical/1 -> Register1/2
  PortAddress/1 -> Relational1/2
  Data/1 -> Register1/1
  PortId/1 -> Relational1/1
  Write/1 -> Logical/2
  Register1/1 -> LatchedData/1

== system N3Z_tonetestprevious/DSProcessor1/OutputRegister/Subsystem7 ==
  Data : Inport
  PortId : Inport  Port=2
  Write : Inport  Port=3
  Logical : xbsIndex_r4/Logical  logical_function=AND  inputs=2  en=off  latency=0  precision=Full  arith_type=Unsigned  n_bits=8  bin_pt=2  align_bp=on  dbl_ovrd=off  block_type=logical
      settings: xl_area=[1 0 0 1 0 0 0]  block_version=VER_STRING_GOES_HERE
  PortAddress : xbsIndex_r4/Constant  const=2  gui_display_data_type=Fixed-point  arith_type=Unsigned  n_bits=8  bin_pt=0  preci_type=Single  exp_width=8  frac_width=24  explicit_period=on  period=fpgaclk  equ=P=C  opselect=C  inp2=PCIN>>17  opr=+  inp1=P  carry=CIN  dbl_ovrd=off  block_type=constant
      settings: block_version=VER_STRING_GOES_HERE
  Register1 : xbsIndex_r4/Register  init=64  rst=off  en=on  dbl_ovrd=off  block_type=register
      settings: xl_area=[4 8 0 0 0 0 0]  block_version=VER_STRING_GOES_HERE
  Relational1 : xbsIndex_r4/Relational  mode=a=b  op_type=Bool  en=off  latency=0  dbl_ovrd=off  block_type=relational
      settings: xl_area=[2 0 0 4 0 0 0]  block_version=VER_STRING_GOES_HERE
  LatchedData : Outport
  wires:
  Relational1/1 -> Logical/1
  Logical/1 -> Register1/2
  PortAddress/1 -> Relational1/2
  Data/1 -> Register1/1
  PortId/1 -> Relational1/1
  Write/1 -> Logical/2
  Register1/1 -> LatchedData/1

== system N3Z_tonetestprevious/DSProcessor1/OutputRegister/Subsystem8 ==
  Data : Inport
  PortId : Inport  Port=2
  Write : Inport  Port=3
  Logical : xbsIndex_r4/Logical  logical_function=AND  inputs=2  en=off  latency=0  precision=Full  arith_type=Unsigned  n_bits=8  bin_pt=2  align_bp=on  dbl_ovrd=off  block_type=logical
      settings: xl_area=[1 0 0 1 0 0 0]  block_version=VER_STRING_GOES_HERE
  PortAddress : xbsIndex_r4/Constant  const=8  gui_display_data_type=Fixed-point  arith_type=Unsigned  n_bits=8  bin_pt=0  preci_type=Single  exp_width=8  frac_width=24  explicit_period=on  period=fpgaclk  equ=P=C  opselect=C  inp2=PCIN>>17  opr=+  inp1=P  carry=CIN  dbl_ovrd=off  block_type=constant
      settings: block_version=VER_STRING_GOES_HERE
  Register1 : xbsIndex_r4/Register  init=0  rst=off  en=on  dbl_ovrd=off  block_type=register
      settings: xl_area=[4 8 0 0 0 0 0]  block_version=VER_STRING_GOES_HERE
  Relational1 : xbsIndex_r4/Relational  mode=a=b  op_type=Bool  en=off  latency=0  dbl_ovrd=off  block_type=relational
      settings: xl_area=[2 0 0 4 0 0 0]  block_version=VER_STRING_GOES_HERE
  LatchedData : Outport
  W : Outport  Port=2
  wires:
  Relational1/1 -> Logical/1
  Logical/1 -> Register1/2, W/1
  PortAddress/1 -> Relational1/2
  Data/1 -> Register1/1
  PortId/1 -> Relational1/1
  Write/1 -> Logical/2
  Register1/1 -> LatchedData/1

== system N3Z_tonetestprevious/DSProcessor1/OutputRegister/Subsystem9 ==
  Data : Inport
  PortId : Inport  Port=2
  Write : Inport  Port=3
  Logical : xbsIndex_r4/Logical  logical_function=AND  inputs=2  en=off  latency=0  precision=Full  arith_type=Unsigned  n_bits=8  bin_pt=2  align_bp=on  dbl_ovrd=off  block_type=logical
      settings: xl_area=[1 0 0 1 0 0 0]  block_version=VER_STRING_GOES_HERE
  PortAddress : xbsIndex_r4/Constant  const=9  gui_display_data_type=Fixed-point  arith_type=Unsigned  n_bits=8  bin_pt=0  preci_type=Single  exp_width=8  frac_width=24  explicit_period=on  period=fpgaclk  equ=P=C  opselect=C  inp2=PCIN>>17  opr=+  inp1=P  carry=CIN  dbl_ovrd=off  block_type=constant
      settings: block_version=VER_STRING_GOES_HERE
  Register1 : xbsIndex_r4/Register  init=0  rst=off  en=on  dbl_ovrd=off  block_type=register
      settings: xl_area=[4 8 0 0 0 0 0]  block_version=VER_STRING_GOES_HERE
  Relational1 : xbsIndex_r4/Relational  mode=a=b  op_type=Bool  en=off  latency=0  dbl_ovrd=off  block_type=relational
      settings: xl_area=[2 0 0 4 0 0 0]  block_version=VER_STRING_GOES_HERE
  LatchedData : Outport
  wires:
  Relational1/1 -> Logical/1
  Logical/1 -> Register1/2
  PortAddress/1 -> Relational1/2
  Data/1 -> Register1/1
  PortId/1 -> Relational1/1
  Write/1 -> Logical/2
  Register1/1 -> LatchedData/1

== system N3Z_tonetestprevious/DemodulationSSB1/AGCandFilter1/Filter1 ==
  note: 16 bit signed input
  note: This bit implements a filter that switches between emphasis and demphasis when RX/TX
  note: Need to get offsets and number of bits correct from simulations!
      | -Done 2/8/15
  note: Assume single clock cycle pulse
  Strobe : Inport
  Input : Inport  Port=2
  Accumulator : xbsIndex_r4/Accumulator  operation=Add  n_bits=18  overflow=Wrap  scale=1  rst=on  hasbypass=off  infoeditControl=reset for floating point data type must be asserted for a minimum of 2 cycles  en=on  latency=0  msb_inp=100  msb=100  lsb=-100  use_behavioral_HDL=on  implementation=Fabric  dbl_ovrd=off  block_type=accum
  AddSub : xbsIndex_r4/AddSub  mode=Addition  use_carryin=off  use_carryout=off  en=off  latency=0  precision=User Defined  arith_type=Unsigned  n_bits=8  bin_pt=0  quantization=Truncate  overflow=Wrap  use_behavioral_HDL=off  hw_selection=Fabric  pipelined=off  dbl_ovrd=off  block_type=addsub
  Concat : xbsIndex_r4/Concat  num_inputs=2  dbl_ovrd=off  block_type=concat
  Concat1 : xbsIndex_r4/Concat  num_inputs=3  dbl_ovrd=off  block_type=concat
  Constant : xbsIndex_r4/Constant  const=0  gui_display_data_type=Fixed-point  arith_type=Unsigned  n_bits=2  bin_pt=0  preci_type=Single  exp_width=8  frac_width=24  explicit_period=on  period=fpgaclk  equ=P=C  opselect=C  inp2=PCIN>>17  opr=+  inp1=P  carry=CIN  dbl_ovrd=off  block_type=constant
  Constant1 : xbsIndex_r4/Constant  const=1  gui_display_data_type=Fixed-point  arith_type=Unsigned  n_bits=1  bin_pt=0  preci_type=Single  exp_width=8  frac_width=24  explicit_period=on  period=fpgaclk  equ=P=C  opselect=C  inp2=PCIN>>17  opr=+  inp1=P  carry=CIN  dbl_ovrd=off  block_type=constant
  Constant2 : xbsIndex_r4/Constant  const=1  gui_display_data_type=Boolean  arith_type=Boolean  n_bits=1  bin_pt=0  preci_type=Single  exp_width=8  frac_width=24  explicit_period=on  period=fpgaclk  equ=P=C  opselect=C  inp2=PCIN>>17  opr=+  inp1=P  carry=CIN  dbl_ovrd=off  block_type=constant
  Constant3 : xbsIndex_r4/Constant  const=0  gui_display_data_type=Fixed-point  arith_type=Signed (2's comp)  n_bits=16  bin_pt=0  preci_type=Single  exp_width=8  frac_width=24  explicit_period=on  period=fpgaclk  equ=P=C  opselect=C  inp2=PCIN>>17  opr=+  inp1=P  carry=CIN  dbl_ovrd=off  block_type=constant
  Constant4 : xbsIndex_r4/Constant  const=0  gui_display_data_type=Boolean  arith_type=Boolean  n_bits=1  bin_pt=0  preci_type=Single  exp_width=8  frac_width=24  explicit_period=on  period=fpgaclk  equ=P=C  opselect=C  inp2=PCIN>>17  opr=+  inp1=P  carry=CIN  dbl_ovrd=off  block_type=constant
  Convert : xbsIndex_r4/Convert  gui_display_data_type=Boolean  arith_type=Boolean  n_bits=16  bin_pt=14  float_type=Single  exp_bits=8  fraction_bits=24  quantization=Truncate  overflow=Wrap  en=off  latency=0  pipeline=off  dbl_ovrd=off  block_type=convert
  Convert1 : xbsIndex_r4/Convert  gui_display_data_type=Boolean  arith_type=Boolean  n_bits=16  bin_pt=14  float_type=Single  exp_bits=8  fraction_bits=24  quantization=Truncate  overflow=Wrap  en=off  latency=0  pipeline=off  dbl_ovrd=off  block_type=convert
  Counter : xbsIndex_r4/Counter  cnt_type=Free Running  cnt_to=Inf  operation=Up  start_count=0  cnt_by_val=1  arith_type=Unsigned  n_bits=8  bin_pt=0  load_pin=off  rst=off  en=on  explicit_period=on  period=fpgaclk  use_behavioral_HDL=off  implementation=Fabric  dbl_ovrd=off  block_type=counter
  Counter1 : xbsIndex_r4/Counter  cnt_type=Free Running  cnt_to=Inf  operation=Up  start_count=0  cnt_by_val=1  arith_type=Unsigned  n_bits=8  bin_pt=0  load_pin=off  rst=on  en=on  explicit_period=on  period=fpgaclk  use_behavioral_HDL=off  implementation=Fabric  dbl_ovrd=off  block_type=counter
  Delay1 : xbsIndex_r4/Delay  rst=off  infoeditControl=Selection of Reset will increase slice count due to use of real FFs and instead of SRLs  en=off  latency=4  reg_retiming=off  dbl_ovrd=off  block_type=delay
  Delay2 : xbsIndex_r4/Delay  rst=off  infoeditControl=Selection of Reset will increase slice count due to use of real FFs and instead of SRLs  en=off  latency=2  reg_retiming=off  dbl_ovrd=off  block_type=delay
  Delay3 : xbsIndex_r4/Delay  rst=off  infoeditControl=Selection of Reset will increase slice count due to use of real FFs and instead of SRLs  en=off  latency=4  reg_retiming=off  dbl_ovrd=off  block_type=delay
  Dual Port RAM : xbsIndex_r4/Dual Port RAM  depth=1024  initVector=[zeros(512,1);FIRRX/4;FIRTX]  distributed_mem=Block RAM  init_a=0  init_b=0  rst_a=off  rst_b=off  en_a=off  en_b=off  latency=1  write_mode_A=Read After Write  write_mode_B=Read After Write  optimize=Area  dbl_ovrd=off  block_type=dpram
  Inverter : xbsIndex_r4/Inverter  en=off  latency=0  dbl_ovrd=off  block_type=inv
  Inverter1 : xbsIndex_r4/Inverter  en=off  latency=0  dbl_ovrd=off  block_type=inv
  Inverter2 : xbsIndex_r4/Inverter  en=off  latency=0  dbl_ovrd=off  block_type=inv
  Latch : MyFunctions/Latch
      link override Set1: const=1  gui_display_data_type=Boolean  arith_type=Boolean  n_bits=1  bin_pt=0  preci_type=Single  exp_width=8  frac_width=24  explicit_period=on  period=fpgaclk  equ=P=C  opselect=C  inp2=PCIN>>17  opr=+  inp1=P  carry=CIN  dbl_ovrd=off
  Logical : xbsIndex_r4/Logical  logical_function=AND  inputs=2  en=off  latency=0  precision=Full  arith_type=Unsigned  n_bits=16  bin_pt=0  align_bp=on  dbl_ovrd=off  block_type=logical
  Monostable : MyFunctions/Monostable
  Monostable1 : MyFunctions/Monostable
  Mult : xbsIndex_r4/Mult  precision=User Defined  arith_type="Signed  (2's comp)"  n_bits=31  bin_pt=0  quantization=Truncate  overflow=Wrap  en=off  latency=3  use_behavioral_HDL=off  opt=Speed  use_embedded=on  optimum_pipeline=off  pipeline=on  dbl_ovrd=off  use_rpm=on  placement_style=Triangular  block_type=mult
  Mux : xbsIndex_r4/Mux  inputs=2  en=off  latency=0  precision=Full  arith_type=Unsigned  n_bits=16  bin_pt=14  quantization=Truncate  overflow=Wrap  dbl_ovrd=off  block_type=mux
  Register : xbsIndex_r4/Register  init=0  rst=off  en=on  dbl_ovrd=off  block_type=register
  Reinterpret2 : xbsIndex_r4/Reinterpret  force_arith_type=on  arith_type="Signed  (2's comp)"  force_bin_pt=on  bin_pt=0  block_type=cast
      settings: block_version=VER_STRING_GOES_HERE
  Reinterpret3 : xbsIndex_r4/Reinterpret  force_arith_type=on  arith_type="Signed  (2's comp)"  force_bin_pt=on  bin_pt=0  block_type=cast
      settings: block_version=VER_STRING_GOES_HERE
  Slice17 : xbsIndex_r4/Slice  nbits=1  boolean_output=off  mode=Upper Bit Location + Width  bit1=0  base1=MSB of Input  bit0=0  base0=LSB of Input  dbl_ovrd=off  block_type=slice
  Slice18 : xbsIndex_r4/Slice  nbits=18  boolean_output=off  mode=Upper Bit Location + Width  bit1=0  base1=MSB of Input  bit0=0  base0=LSB of Input  dbl_ovrd=off  block_type=slice
  Slice19 : xbsIndex_r4/Slice  nbits=18  boolean_output=off  mode=Upper Bit Location + Width  bit1=0  base1=MSB of Input  bit0=0  base0=LSB of Input  dbl_ovrd=off  block_type=slice
  Output : Outport
  wires:
  Reinterpret3/1 -> Register/1
  Reinterpret2/1 -> Accumulator/1
  Convert1/1 -> Latch/2
  Input/1 -> Dual Port RAM/2
  Register/1 -> Output/1
  Strobe/1 -> Convert/1
  AddSub/1 -> Mux/3
  Slice19/1 -> Reinterpret3/1
  Slice18/1 -> Reinterpret2/1
  Dual Port RAM/2 -> Mult/2
  Dual Port RAM/1 -> Mult/1
  Monostable1/1 -> Register/2, Accumulator/2
  Inverter2/1 -> Monostable1/1
  Accumulator/1 -> Slice19/1
  Mult/1 -> Slice18/1
  Delay3/1 -> Accumulator/3, Inverter2/1
  Monostable/1 -> Convert1/1
  Inverter1/1 -> Monostable/1
  Slice17/1 -> Inverter1/1
  Delay2/1 -> Counter1/2
  Convert/1 -> Counter/1, Delay1/1, Logical/2
  Constant4/1 -> Dual Port RAM/6
  Constant3/1 -> Dual Port RAM/5
  Mux/1 -> Concat/2
  Counter/1 -> Mux/2, AddSub/1
  Concat/1 -> Dual Port RAM/1
  Inverter/1 -> Counter1/1
  Latch/1 -> Mux/1, Inverter/1, Delay2/1, Delay3/1
  Delay1/1 -> Latch/1
  Logical/1 -> Dual Port RAM/3
  Constant2/1 -> Logical/1
  Concat1/1 -> Dual Port RAM/4
  Counter1/1 -> Concat1/3, AddSub/2, Slice17/1
  Constant1/1 -> Concat1/1
  [TX_High] -> Concat1/2
  Constant/1 -> Concat/1

== system N3Z_tonetestprevious/DemodulationSSB1/FilterStreamIntegration/TrigDistrib ==
  Trig : Inport
  In2 : Inport  Port=2
  3LineTo8Way : Subsystem
  Logical{,1..7} (8 alike) : xbsIndex_r4/Logical  logical_function=AND  inputs=2  en=off  latency=0  precision=Full  arith_type=Unsigned  n_bits=16  bin_pt=0  align_bp=on  dbl_ovrd=off  block_type=logical
      settings: xl_area=[1 0 0 1 0 0 0]  block_version=8.2.02
  Out1 : Outport
  Out2 : Outport  Port=2
  Out3 : Outport  Port=3
  Out4 : Outport  Port=4
  Out5 : Outport  Port=5
  Out6 : Outport  Port=6
  Out7 : Outport  Port=7
  Out8 : Outport  Port=8
  wires:
  Trig/1 -> Logical/1, Logical1/1, Logical2/1, Logical3/1, Logical4/1, Logical5/1, Logical6/1, Logical7/1
  3LineTo8Way/1(Out1) -> Logical/2
  3LineTo8Way/2(Out2) -> Logical1/2
  3LineTo8Way/3(Out3) -> Logical2/2
  3LineTo8Way/4(Out4) -> Logical3/2
  3LineTo8Way/5(Out5) -> Logical4/2
  3LineTo8Way/6(Out6) -> Logical5/2
  3LineTo8Way/7(Out7) -> Logical6/2
  3LineTo8Way/8(Out8) -> Logical7/2
  Logical/1 -> Out1/1
  Logical1/1 -> Out2/1
  In2/1 -> 3LineTo8Way/1(In1)
  Logical2/1 -> Out3/1
  Logical3/1 -> Out4/1
  Logical4/1 -> Out5/1
  Logical5/1 -> Out6/1
  Logical6/1 -> Out7/1
  Logical7/1 -> Out8/1

== system N3Z_tonetestprevious/DemodulationSSB1/FilterStreamIntegration/TrigDistrib1 ==
  Trig : Inport
  In2 : Inport  Port=2
  3LineTo8Way : Subsystem
  Logical{,1..7} (8 alike) : xbsIndex_r4/Logical  logical_function=AND  inputs=2  en=off  latency=0  precision=Full  arith_type=Unsigned  n_bits=16  bin_pt=0  align_bp=on  dbl_ovrd=off  block_type=logical
      settings: xl_area=[1 0 0 1 0 0 0]  block_version=8.2.02
  Out1 : Outport
  Out2 : Outport  Port=2
  Out3 : Outport  Port=3
  Out4 : Outport  Port=4
  Out5 : Outport  Port=5
  Out6 : Outport  Port=6
  Out7 : Outport  Port=7
  Out8 : Outport  Port=8
  wires:
  Trig/1 -> Logical/1, Logical1/1, Logical2/1, Logical3/1, Logical4/1, Logical5/1, Logical6/1, Logical7/1
  3LineTo8Way/1(Out1) -> Logical/2
  3LineTo8Way/2(Out2) -> Logical1/2
  3LineTo8Way/3(Out3) -> Logical2/2
  3LineTo8Way/4(Out4) -> Logical3/2
  3LineTo8Way/5(Out5) -> Logical4/2
  3LineTo8Way/6(Out6) -> Logical5/2
  3LineTo8Way/7(Out7) -> Logical6/2
  3LineTo8Way/8(Out8) -> Logical7/2
  Logical/1 -> Out1/1
  Logical1/1 -> Out2/1
  In2/1 -> 3LineTo8Way/1(In1)
  Logical2/1 -> Out3/1
  Logical3/1 -> Out4/1
  Logical4/1 -> Out5/1
  Logical5/1 -> Out6/1
  Logical6/1 -> Out7/1
  Logical7/1 -> Out8/1

== system N3Z_tonetestprevious/KeyPadinterface/OutputRegister/Subsystem1 ==
  Data : Inport
  PortId : Inport  Port=2
  Write : Inport  Port=3
  Logical : xbsIndex_r4/Logical  logical_function=AND  inputs=2  en=off  latency=0  precision=Full  arith_type=Unsigned  n_bits=8  bin_pt=2  align_bp=on  dbl_ovrd=off  block_type=logical
      settings: xl_area=[1 0 0 1 0 0 0]  block_version=VER_STRING_GOES_HERE
  PortAddress : xbsIndex_r4/Constant  const=5  gui_display_data_type=Fixed-point  arith_type=Unsigned  n_bits=8  bin_pt=0  preci_type=Single  exp_width=8  frac_width=24  explicit_period=on  period=fpgaclk  equ=P=C  opselect=C  inp2=PCIN>>17  opr=+  inp1=P  carry=CIN  dbl_ovrd=off  block_type=constant
      settings: block_version=VER_STRING_GOES_HERE
  Register1 : xbsIndex_r4/Register  init=0  rst=off  en=on  dbl_ovrd=off  block_type=register
      settings: xl_area=[4 8 0 0 0 0 0]  block_version=VER_STRING_GOES_HERE
  Relational1 : xbsIndex_r4/Relational  mode=a=b  op_type=Bool  en=off  latency=0  dbl_ovrd=off  block_type=relational
      settings: xl_area=[2 0 0 4 0 0 0]  block_version=VER_STRING_GOES_HERE
  LatchedData : Outport
  Strobe : Outport  Port=2
  wires:
  Relational1/1 -> Logical/1
  Logical/1 -> Register1/2, Strobe/1
  PortAddress/1 -> Relational1/2
  Data/1 -> Register1/1
  PortId/1 -> Relational1/1
  Write/1 -> Logical/2
  Register1/1 -> LatchedData/1
